simulink model "BLDC_block_commutation1"  (R2012b)
settings: Solver=ode45  StartTime=0.0  StopTime=1  RelTol=1e-3
libraries: BLDC x1
settings Model: Creator=h3now  LastModifiedBy=h3now

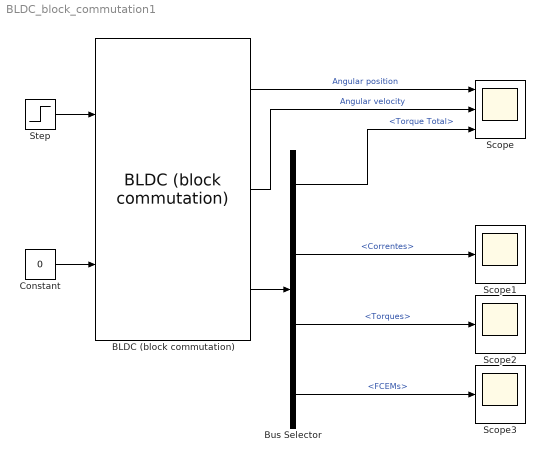
== system BLDC_block_commutation1 ==
  BLDC (block commutation) : BLDC/BLDC (block commutation)  J=1.39e-6  R=10.1/2  L=2.04/2000  P=8  Kt=15.7e-3/1.19  Ke=15.7e-3/1.19  Kd=0
  Bus Selector : BusSelector  OutputSignals=Torque Total,Correntes,Torques,FCEMs
  Constant : Constant  Value=0
  Scope : Scope  NumInputPorts=3
      settings: ShowLegends=on  YMin=-5~-5~-5  YMax=5~5~5
  Scope1 : Scope
  Scope2 : Scope
      settings: SaveName=ScopeData2
  Scope3 : Scope
      settings: SaveName=ScopeData3
  Step : Step  Time=0  After=12  SampleTime=0
  wires:
  BLDC (block commutation)/1 -> Scope/1  "Angular position"
  Step/1 -> BLDC (block commutation)/1
  Constant/1 -> BLDC (block commutation)/2
  BLDC (block commutation)/2 -> Scope/2  "Angular velocity"
  BLDC (block commutation)/3 -> Bus Selector/1
  Bus Selector/1 -> Scope/3  "<Torque Total>"
  Bus Selector/2 -> Scope1/1  "<Correntes>"
  Bus Selector/3 -> Scope2/1  "<Torques>"
  Bus Selector/4 -> Scope3/1  "<FCEMs>"
